simulink model "Task4"  (R2022a)
settings: Solver=FixedStepAuto  StartTime=0.0  StopTime=10.0  FixedStep=0.0001  RelTol=1e-3
undefined symbols (not defined in the file): K, T1, T2
settings Model: Creator=Family  LastModifiedBy=Family

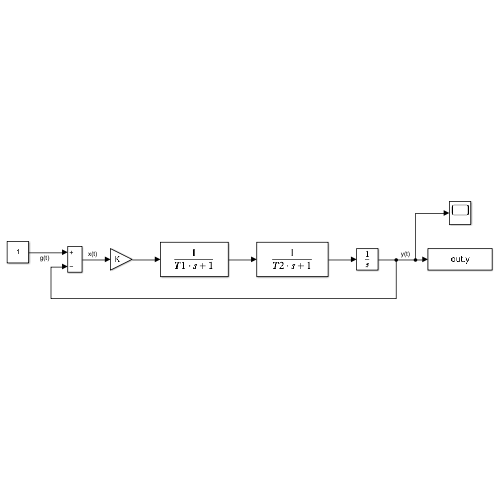
[thumbnail: Simulink's stored preview of the top-level diagram]
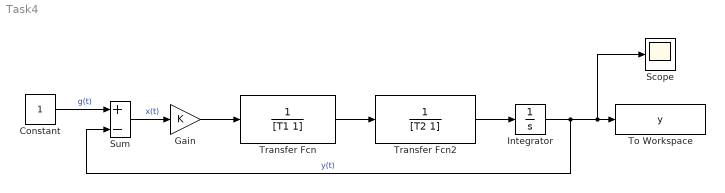
== system Task4 ==
  Constant : Constant
  Gain : Gain  Gain=K
  Integrator : Integrator
  Scope : Scope
  Sum : Sum  Inputs=+-
  To Workspace : ToWorkspace  VariableName=y  SaveFormat=Timeseries  SampleTime=-1
  Transfer Fcn : TransferFcn  Denominator=[T1 1]
  Transfer Fcn2 : TransferFcn  Denominator=[T2 1]
  wires:
  Integrator/1 -> Scope/1, To Workspace/1, Sum/2  "y(t)"
  Transfer Fcn/1 -> Transfer Fcn2/1
  Sum/1 -> Gain/1  "x(t)"
  Gain/1 -> Transfer Fcn/1
  Transfer Fcn2/1 -> Integrator/1
  Constant/1 -> Sum/1  "g(t)"
